simulink library "PID_discrete_block"  (Simulink 2.20)

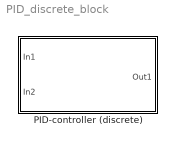
== system PID_discrete_block ==
  PID-controller (discrete) : Subsystem  Description=PID_regulator  mask(PID_regulator){P=1, I=1, D=1, T=1}
      mask prompts: P "P="; I "I="; D "D="; T "T="
      mask help: PID discrete controller
      mask init:
      | q2=P*D/T;
      | q0=P+q2;
      | q1=-P+P*T/I-2*q2;
      mask Help: enter P,I,D,T

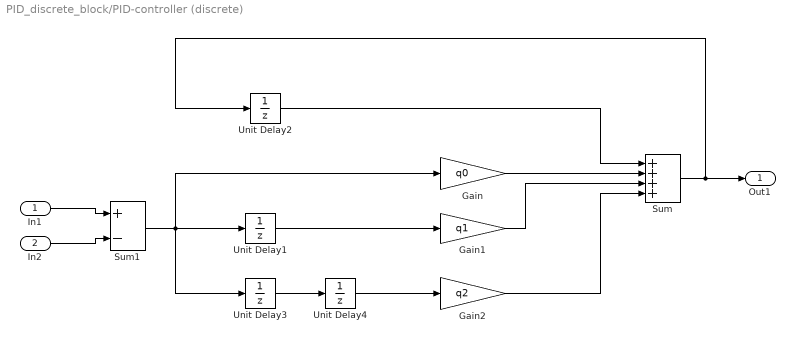
== system PID_discrete_block/PID-controller (discrete) ==
  In1 : Inport  Port=1  PortWidth=-1  SampleTime=-1
  In2 : Inport  Port=2  PortWidth=-1  SampleTime=-1
  Gain : Gain  Gain=q0
  Gain1 : Gain  Gain=q1
  Gain2 : Gain  Gain=q2
  Sum : Sum  Inputs=++++
  Sum1 : Sum  Inputs=+-
  Unit Delay{1..4} (4 alike) : UnitDelay  X0=0  SampleTime=1
  Out1 : Outport  Port=1
  wires:
  Gain2/1 -> Sum/4
  Unit Delay2/1 -> Sum/1
  Gain1/1 -> Sum/3
  Gain/1 -> Sum/2
  Sum1/1 -> Gain/1, Unit Delay1/1, Unit Delay3/1
  Unit Delay4/1 -> Gain2/1
  Unit Delay3/1 -> Unit Delay4/1
  Unit Delay1/1 -> Gain1/1
  Sum/1 -> Unit Delay2/1, Out1/1
  In1/1 -> Sum1/1
  In2/1 -> Sum1/2
